simulink model "ugrid_hdetail_mod_linea_transmision"  (R2018a)
settings: Solver=VariableStepAuto  StartTime=0.0  StopTime=1  FixedStep=1e-6  MaxStep=1e-4  RelTol=1e-3
InitFcn:
  | SimulinkInit_linea_transmision
values from neighbouring files (symbols this model uses):
  b = 4.91    [SimulinkInit_linea_transmision.m]    (also in parametros_BIO.m; sistema.m = num(2))
  C = [C11; C22; C33;C44]    [Parametros_Sistema.m]    (also in SimulinkInit.m = 0.002654; SimulinkInit_linea_transmision.m = 1)
  C1 = 22e-6    (= 2.2e-05)    [Parametros_Sistema.m]    (also in SimulinkInit.m; SimulinkInit_linea_transmision.m; sistema.m)
  C2 = 22e-6    (= 2.2e-05)    [Parametros_Sistema.m]    (also in SimulinkInit.m; SimulinkInit_linea_transmision.m; sistema.m)
  C3 = 610e-6    (= 0.00061)    [Parametros_Sistema.m]    (also in SimulinkInit.m; SimulinkInit_linea_transmision.m; sistema.m)
  Cl = 20000e-6    (= 0.02)    [Parametros_Sistema.m]    (also in SimulinkInit.m = 0.002; SimulinkInit_linea_transmision.m; sistema.m)
  K = 25    [SimulinkInit_linea_transmision.m]    (also in parametros_BIO.m)
  K1 = 1.15    [SimulinkInit.m]    (also in SimulinkInit_linea_transmision.m = 9.66)
  K11 = 0.8    [SimulinkInit_linea_transmision.m]    (also in parametros_BIO.m)
  K2 = 1    [SimulinkInit.m]    (also in SimulinkInit_linea_transmision.m = 6.97)
  K22 = 0.2    [SimulinkInit_linea_transmision.m]    (also in parametros_BIO.m)
  K3 = 1    [SimulinkInit.m]    (also in SimulinkInit_linea_transmision.m = 31.8)
  K33 = 0.23    [SimulinkInit_linea_transmision.m]    (also in parametros_BIO.m)
  K4 = 15.1    [SimulinkInit_linea_transmision.m]    (also in parametros_BIO.m)
  Kd = 0.02    [SimulinkInit_linea_transmision.m]    (also in parametros_BIO.m)
  Kdc = 0.02    [SimulinkInit_linea_transmision.m]    (also in parametros_BIO.m)
  Kf = 1    [SimulinkInit_linea_transmision.m]    (also in parametros_BIO.m)
  Kh = 1.2    [SimulinkInit_linea_transmision.m]    (also in parametros_BIO.m)
  Ks = 21.5    [SimulinkInit_linea_transmision.m]    (also in parametros_BIO.m)
  Ksc = 3    [SimulinkInit_linea_transmision.m]    (also in parametros_BIO.m)
  Kv = 1    [SimulinkInit_linea_transmision.m]    (also in parametros_BIO.m)
  L = 5.2    [Parametros_Sistema.m]    (also in SimulinkInit_linea_transmision.m; sistema.m)
  L1 = 40e-3    (= 0.04)    [Parametros_Sistema.m]    (also in SimulinkInit.m; SimulinkInit_linea_transmision.m; sistema.m)
  L2 = 30e-3    (= 0.03)    [Parametros_Sistema.m]    (also in SimulinkInit.m = 0.005; SimulinkInit_linea_transmision.m; sistema.m)
  L3 = 5e-3    (= 0.005)    [Parametros_Sistema.m]    (also in SimulinkInit.m = 0.03; SimulinkInit_linea_transmision.m; sistema.m)
  L4 = 1e-3    (= 0.001)    [Parametros_Sistema.m]    (also in SimulinkInit.m = 5.2; SimulinkInit_linea_transmision.m = 3.5e-05; sistema.m)
  L5 = 10e-3    (= 0.01)    [Parametros_Sistema.m]    (also in SimulinkInit_linea_transmision.m = 2.2e-05; sistema.m)
  L6 = 40e-3    (= 0.04)    [Parametros_Sistema.m]    (also in SimulinkInit_linea_transmision.m = 1e-05; sistema.m)
  R = 10    [Parametros_Sistema.m]    (also in SimulinkInit_linea_transmision.m; sistema.m)
  R1 = 0.1    [Parametros_Sistema.m]    (also in SimulinkInit.m; SimulinkInit_linea_transmision.m; sistema.m)
  R2 = 0.2    [Parametros_Sistema.m]    (also in SimulinkInit.m = 0.1; SimulinkInit_linea_transmision.m; sistema.m)
  R3 = 1e-3    (= 0.001)    [Parametros_Sistema.m]    (also in SimulinkInit.m; SimulinkInit_linea_transmision.m; sistema.m)
  R4 = 10    [Parametros_Sistema.m]    (also in SimulinkInit.m; SimulinkInit_linea_transmision.m = 0.005; sistema.m)
  R5 = 4    [Parametros_Sistema.m]    (also in SimulinkInit.m = 10; SimulinkInit_linea_transmision.m = 0.0012; sistema.m)
  R6 = 25    [Parametros_Sistema.m]    (also in SimulinkInit_linea_transmision.m = 0.001; sistema.m)
  RL = 10    [Parametros_Sistema.m]    (also in SimulinkInit_linea_transmision.m; sistema.m)
  Sbin = 13.8    [SimulinkInit_linea_transmision.m]    (also in parametros_BIO.m)
  Svin = 2.91    [SimulinkInit_linea_transmision.m]    (also in parametros_BIO.m)
  T1 = 0.4    [SimulinkInit_linea_transmision.m]    (also in parametros_BIO.m)
  T2 = 1    [SimulinkInit_linea_transmision.m]    (also in parametros_BIO.m)
  T3 = 15    [SimulinkInit_linea_transmision.m]    (also in parametros_BIO.m)
  T4 = 2.5    [SimulinkInit_linea_transmision.m]    (also in parametros_BIO.m)
  T5 = 3.3    [SimulinkInit_linea_transmision.m]    (also in parametros_BIO.m)
  Tao1 = 0.5    [SimulinkInit.m]
  Tcd = 0.2    [SimulinkInit_linea_transmision.m]    (also in parametros_BIO.m)
  Tcr = 0.01    [SimulinkInit_linea_transmision.m]    (also in parametros_BIO.m)
  Tf = 0.04    [SimulinkInit_linea_transmision.m]    (also in parametros_BIO.m)
  Tr = 950    [SimulinkInit_linea_transmision.m]    (also in parametros_BIO.m)
  Tt = 450    [SimulinkInit_linea_transmision.m]    (also in parametros_BIO.m)
  Ttd = 0.04    [SimulinkInit_linea_transmision.m]    (also in parametros_BIO.m)
  Tv = 0.05    [SimulinkInit_linea_transmision.m]    (also in parametros_BIO.m)
  V = 20    [SimulinkInit_linea_transmision.m]    (also in parametros_BIO.m)
  wref = 70000    [SimulinkInit_linea_transmision.m]    (also in parametros_BIO.m)
  X_acid = 1.2    [SimulinkInit_linea_transmision.m]    (also in parametros_BIO.m)
  X_meth = 0.35    [SimulinkInit_linea_transmision.m]    (also in parametros_BIO.m)
  Z = 3    [SimulinkInit_linea_transmision.m]    (also in parametros_BIO.m)
undefined symbols (not defined in the file or in its folder): Ion, Lithium, sigbuilder_block, ss1, ss2
libraries: powerlib x64, dsparch4 x18, powerlib_meascontrol x4, simulink x1, mpclib x1, electricdrivelib x1
(part 2 of 2)

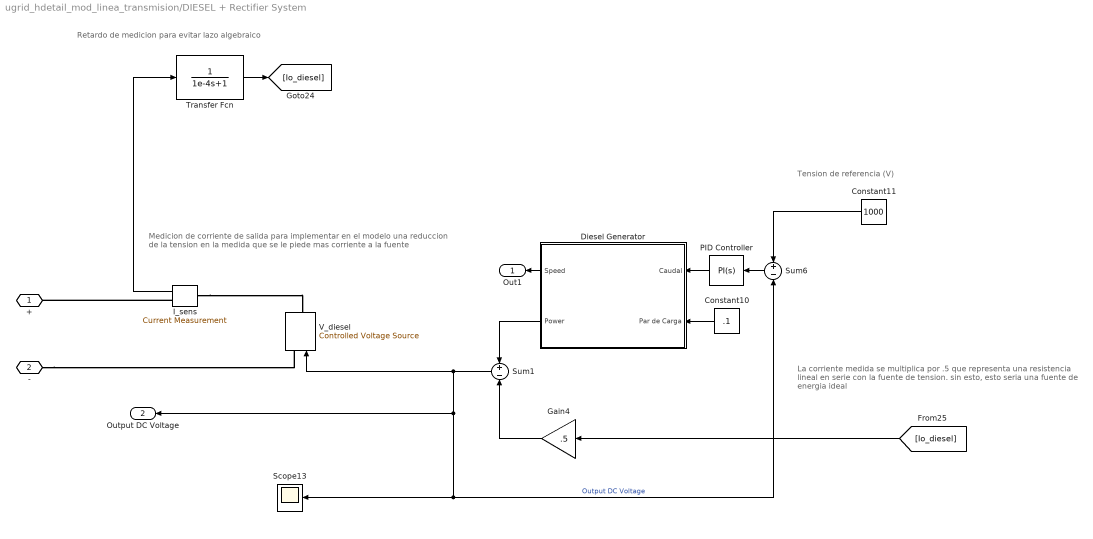
== system ugrid_hdetail_mod_linea_transmision/DIESEL + Rectifier System ==
  note: Tension de referencia (V)
  note: La corriente medida se multiplica por .5 que
      | representa una resistencia lineal en serie con
      | la fuente de tension. sin esto, esto seria una
      | fuente de energia ideal
  note: Medicion de corriente de salida para implementar
      | en el modelo una reduccion de la tension en la
      | medida que se le piede mas corriente a la fuente
  note: Retardo de medicion para evitar lazo algebraico
  Constant10 : Constant  Value=.1
  Constant11 : Constant  Value=1000
  Diesel Generator : Subsystem
  Gain4 : Gain  Gain=.5
  I_sens : powerlib/Measurements/Current Measurement  PhasorSimulation=off  OutputType=Complex  PSBequivalent=0
  PID Controller : simulink/Continuous/PID Controller  Controller=PI  TimeDomain=Continuous-time  SampleTime=-1  IntegratorMethod=Forward Euler  FilterMethod=Forward Euler  Form=Parallel  UseFilter=on  ControllerParametersSource=internal  P=0.00325909628031494  I=0.000326732379168699  D=0.00124823483730586  N=0.606508283225141  InitialConditionSource=internal  InitialConditionForIntegrator=0.248  InitialConditionForFilter=0.24  ExternalReset=none  LimitOutput=off  UpperSaturationLimit=inf  LowerSaturationLimit=-inf  LinearizeAsGain=on  AntiWindupMode=none  Kb=1  TrackingMode=off  Kt=1  PParamMin=[]  PParamMax=[]  IParamMin=[]  IParamMax=[]  DParamMin=[]  DParamMax=[]  NParamMin=[]  NParamMax=[]  KbParamMin=[]  KbParamMax=[]  KtParamMin=[]  KtParamMax=[]  POutMin=[]  POutMax=[]  IOutMin=[]  IOutMax=[]  DOutMin=[]  DOutMax=[]  NOutMin=[]  NOutMax=[]  KbOutMin=[]  KbOutMax=[]  KtOutMin=[]  KtOutMax=[]  IntegratorOutMin=[]  IntegratorOutMax=[]  FilterOutMin=[]  FilterOutMax=[]  SumOutMin=[]  SumOutMax=[]  SumI1OutMin=[]  SumI1OutMax=[]  SumI2OutMin=[]  SumI2OutMax=[]  SumI3OutMin=[]  SumI3OutMax=[]  SumDOutMin=[]  SumDOutMax=[]  SaturationOutMin=[]  SaturationOutMax=[]  IntegratorContinuousStateAttributes=''  IntegratorStateMustResolveToSignalObject=off  IntegratorRTWStateStorageClass=Auto  FilterContinuousStateAttributes=''  FilterStateMustResolveToSignalObject=off  FilterRTWStateStorageClass=Auto  DifferentiatorICPrevScaledInput=0  DifferentiatorOutMin=[]  DifferentiatorOutMax=[]  InitialConditionSetting=State (most efficient)  FilterDiffOutCoefMin=[]  FilterDiffOutCoefMax=[]  SumDenOutMin=[]  SumDenOutMax=[]  SumNumOutMin=[]  SumNumOutMax=[]  ReciprocalOutMin=[]  ReciprocalOutMax=[]  DivideOutMin=[]  DivideOutMax=[]  TunerSelectOption=Transfer Function Based (PID Tuner App)
  Scope13 : Scope
  Sum1 : Sum  Inputs=+-
  Sum6 : Sum  Inputs=+-
  Transfer Fcn : TransferFcn  Denominator=[1e-4 1]
  V_diesel : powerlib/Electrical Sources/Controlled Voltage Source  Initialize=on  Source_Type=AC  Amplitude=0  Phase=0  Frequency=0  Measurements=None
  + : PMIOPort  Side=Left
  - : PMIOPort  Port=2  Side=Left
  Out1 : Outport
  Output DC Voltage : Outport  Port=2
  wires:
  Sum1/1 -> Output DC Voltage/1, Sum6/2, Scope13/1, V_diesel/1  "Output DC Voltage"
  Transfer Fcn/1 -> [Io_diesel]
  I_sens/1 -> Transfer Fcn/1
  Diesel Generator/2(Power) -> Sum1/1
  Sum6/1 -> PID Controller/1
  Diesel Generator/1(Speed) -> Out1/1
  Gain4/1 -> Sum1/2
  Constant10/1 -> Diesel Generator/2(Par de Carga)
  Constant11/1 -> Sum6/1
  [Io_diesel] -> Gain4/1
  PID Controller/1 -> Diesel Generator/1(Caudal)
  connections:
  -/RConn1 -- V_diesel/LConn1
  I_sens/LConn1 -- V_diesel/RConn1
  I_sens/RConn1 -- +/RConn1

== system ugrid_hdetail_mod_linea_transmision/Signal Builder ==
  Demux : Demux  Tag=STV Demux  Outputs=1
  FromWs : FromWorkspace  Tag=STV FromWs  VariableName=tuvar  SampleTime=0
      SigBuilderData=|
      | common.afterFinalStr = 'Extrapolate'
      | common.sampleTime = 0
      | dataSet.timeRange = [0 10]
      | dataSet.name = 'Group 1'
      | sbobj.Groups.Name = 'Group 1'
      | sbobj.Groups.Signals.Name = 'Signal 1'
      | sbobj.Groups.Signals.XData = [0 0.1 0.1 0.2 0.2 0.3 0.3 0.4 0.4 0.5 0.5 0.6 0.6 0.7 0.7 0.8 0.8 0.9 0.9 10]
      | sbobj.Groups.Signals.YData = [0 0 500 500 1000 1000 1500 1500 2000 2000 2500 2500 3000 3000 3500 3500 4000 4000 4500 4500]
  Signal 1 : Outport  Tag=STV Outport
  wires:
  Demux/1 -> Signal 1/1
  FromWs/1 -> Demux/1

== system ugrid_hdetail_mod_linea_transmision/Signal Builder1 ==
  Demux : Demux  Tag=STV Demux  Outputs=1
  FromWs : FromWorkspace  Tag=STV FromWs  VariableName=tuvar  SampleTime=0
      SigBuilderData=|
      | common.afterFinalStr = 'Extrapolate'
      | common.sampleTime = 0
      | dataSet.timeRange = [0 10]
      | dataSet.name = 'Group 1'
      | sbobj.Groups.Name = 'Group 1'
      | sbobj.Groups.Signals.Name = 'Signal 1'
      | sbobj.Groups.Signals.XData = [0 0.1 0.1 0.4 0.4 0.8 0.8 10]
      | sbobj.Groups.Signals.YData = [0 0 100 100 200 200 500 500]
  Signal 1 : Outport  Tag=STV Outport
  wires:
  FromWs/1 -> Demux/1
  Demux/1 -> Signal 1/1

== system ugrid_hdetail_mod_linea_transmision/Signal Builder2 ==
  Demux : Demux  Tag=STV Demux  Outputs=1
  FromWs : FromWorkspace  Tag=STV FromWs  VariableName=tuvar  SampleTime=0
      SigBuilderData=|
      | common.afterFinalStr = 'Extrapolate'
      | common.sampleTime = 0
      | dataSet.timeRange = [0 10]
      | dataSet.name = 'Group 1'
      | sbobj.Groups.Name = 'Group 1'
      | sbobj.Groups.Signals.Name = 'Signal 1'
      | sbobj.Groups.Signals.XData = [0 0.1 0.1 0.2 0.2 0.3 0.3 0.4 0.4 0.5 0.5 0.6 0.6 0.7 0.7 0.8 0.8 0.9 0.9 10]
      | sbobj.Groups.Signals.YData = [0 0 500 500 1000 1000 1500 1500 2000 2000 2500 2500 3000 3000 3500 3500 4000 4000 4500 4500]
  Signal 1 : Outport  Tag=STV Outport
  wires:
  FromWs/1 -> Demux/1
  Demux/1 -> Signal 1/1

== system ugrid_hdetail_mod_linea_transmision/Signal Builder3 ==
  Demux : Demux  Tag=STV Demux  Outputs=1
  FromWs : FromWorkspace  Tag=STV FromWs  VariableName=tuvar  SampleTime=0
      SigBuilderData=|
      | common.afterFinalStr = 'Extrapolate'
      | common.sampleTime = 0
      | dataSet.timeRange = [0 10]
      | dataSet.name = 'Group 1'
      | sbobj.Groups.Name = 'Group 1'
      | sbobj.Groups.Signals.Name = 'Signal 1'
      | sbobj.Groups.Signals.XData = [0 0.1 0.1 0.4 0.4 0.8 0.8 10]
      | sbobj.Groups.Signals.YData = [0 0 100 100 200 200 500 500]
  Signal 1 : Outport  Tag=STV Outport
  wires:
  Demux/1 -> Signal 1/1
  FromWs/1 -> Demux/1

== system ugrid_hdetail_mod_linea_transmision/Subsystem ==
  Battery : electricdrivelib/Extra Sources/Battery  BatType=Lithium-Ion  ShowTempParam=off  ThermalPreset=no  ShowAgeParam=off  NomV=1000  NomQ=20  SOC=100  Batt_Tr=10e-3  PresetModel=off  MaxQ=1  MinV=825  FullV=1280.3859  Dis_rate=200  R=50e-3  Normal_OP=0.90435  expZone="[1188.4244    0.049130435]"  current=[6.5 13 32.5 50]  Units=Time  Tci=20  NomT=20  T2=-30  MaxQ2=4.8  FullV2=7.1  Normal_OP2=5.655  expZone2="[6.58           1]"  Rca=0.6  ti=2000  Dp=0  Neq0=0  Tsim=1e6  Ta1=25  Qeol=5.4*0.9  Reol=0.013333*1.2  Char_age=[2.3478, 3]  Dis_age=[2.3478, 10]  N1=1500  N2=10500  N3=1000  N4=1400  Ta2=45  N5=950
  Constant2 : Constant  Value=1000
  Constant4 : Constant  Value=25
  Controlled Current Source : powerlib/Electrical Sources/Controlled Current Source  Initialize=on  Source_Type=AC  Amplitude=0  Phase=0  Frequency=0  Measurements=None
  Gain3 : Gain  Gain=1/10
  PV panel1 : Subsystem
      mask Display: image('panel.jpg')
  Rcable : powerlib/Elements/Series RLC Branch  LConnTagsString=__new0  RConnTagsString=__new0  BranchType=R  Resistance=1e-3  Inductance=1e-3  SetiL0=off  InitialCurrent=0  Capacitance=1e-6  Setx0=off  InitialVoltage=0  Measurements=None
  Rin2 : powerlib/Elements/Series RLC Branch  LConnTagsString=__new0  RConnTagsString=__new0  BranchType=C  Resistance=.001  Inductance=0  SetiL0=off  InitialCurrent=0  Capacitance=1000e-6  Setx0=off  InitialVoltage=0  Measurements=None
  + : PMIOPort  Side=Left
  - : PMIOPort  Port=2  Side=Left
  Out1 : Outport
  wires:
  PV panel1/1(I) -> Gain3/1
  Gain3/1 -> Controlled Current Source/1
  Battery/1 -> Out1/1
  Constant4/1 -> PV panel1/3(Top)
  Constant2/1 -> PV panel1/2(G)
  [V] -> PV panel1/1(V)
  connections:
  Rcable/RConn1 -- +/RConn1
  Battery/LConn1 -- Controlled Current Source/RConn1 -- Rcable/LConn1 -- Rin2/LConn1
  Battery/LConn2 -- -/RConn1 -- Rin2/RConn1 -- Controlled Current Source/LConn1

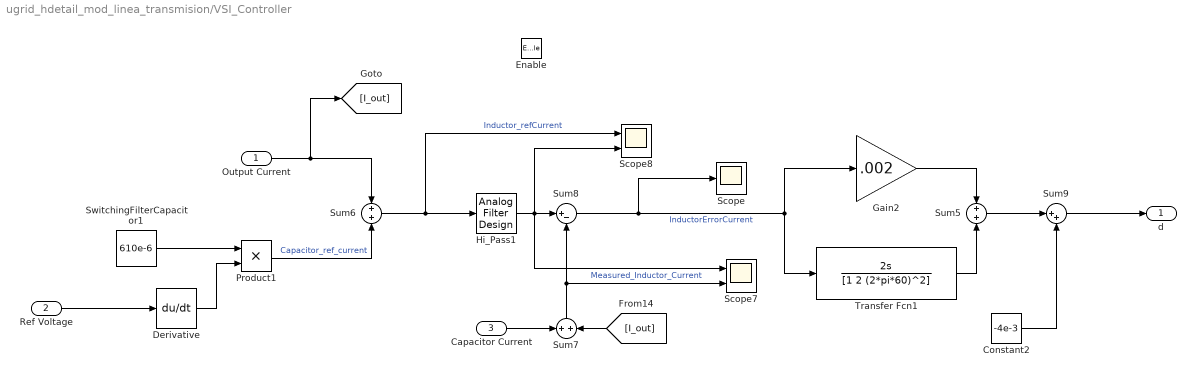
== system ugrid_hdetail_mod_linea_transmision/VSI_Controller ==
  Output Current : Inport
  Ref Voltage : Inport  Port=2
  Capacitor Current : Inport  Port=3
  Enable : EnablePort
  Constant2 : Constant  Value=-4e-3
  Derivative : Derivative  CoefficientInTFapproximation=1e-3
  Gain2 : Gain  Gain=.002
  Hi_Pass1 : dsparch4/Analog Filter Design  method=Bessel  filttype=Highpass  N=1  Wlo=1*2*pi  Whi=80  Rp=2  Rs=40
  Product1 : Product
  Scope : Scope
  Scope7 : Scope  NumInputPorts=2
  Scope8 : Scope  NumInputPorts=2
  Sum5 : Sum  Inputs=+|+
  Sum6 : Sum  Inputs=+|+
  Sum7 : Sum  Inputs=+|+
  Sum8 : Sum  Inputs=|+-
  Sum9 : Sum  Inputs=|++
  SwitchingFilterCapacitor1 : Constant  Value=610e-6
  Transfer Fcn1 : TransferFcn  Numerator=[2 0]  Denominator=[1 2 (2*pi*60)^2]
  d : Outport
  wires:
  Derivative/1 -> Product1/2
  Sum6/1 -> Hi_Pass1/1, Scope8/1  "Inductor_refCurrent"
  Sum8/1 -> Scope/1, Transfer Fcn1/1, Gain2/1  "InductorErrorCurrent"
  Ref Voltage/1 -> Derivative/1
  Constant2/1 -> Sum9/2
  Capacitor Current/1 -> Sum7/1
  Transfer Fcn1/1 -> Sum5/2
  Output Current/1 -> Sum6/1, [I_out]
  [I_out] -> Sum7/2
  Gain2/1 -> Sum5/1
  SwitchingFilterCapacitor1/1 -> Product1/1
  Hi_Pass1/1 -> Scope8/2, Sum8/1, Scope7/1
  Product1/1 -> Sum6/2  "Capacitor_ref_current"
  Sum9/1 -> d/1
  Sum5/1 -> Sum9/1
  Sum7/1 -> Scope7/2, Sum8/2  "Measured_Inductor_Current"

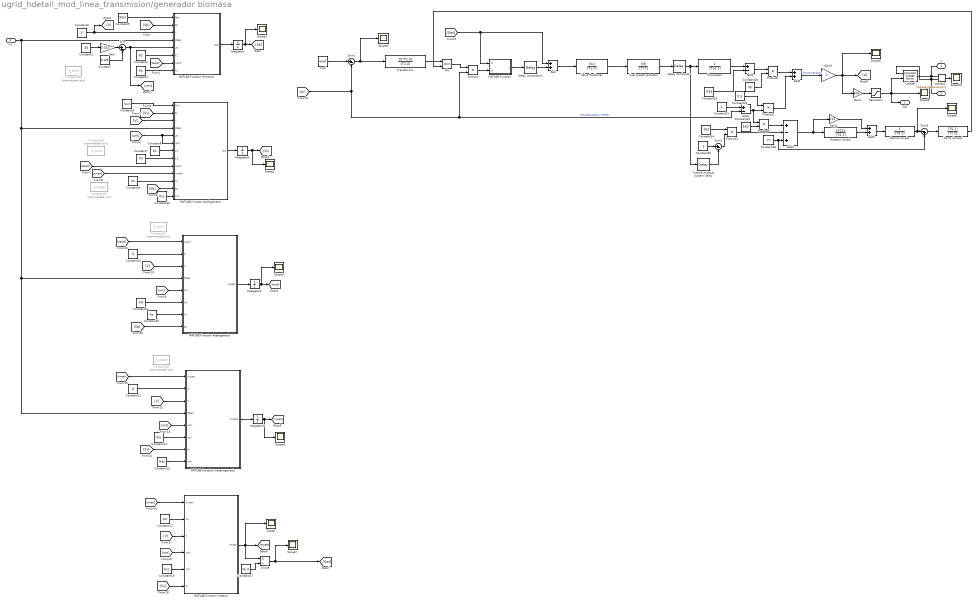
== system ugrid_hdetail_mod_linea_transmision/generador biomasa ==
  In1 : Inport
  Add : Sum
  Add1 : Sum  Inputs=+-
  Add2 : Sum
  Add3 : Sum  Inputs=+-
  Add4 : Sum  Inputs=+-+
  Add5 : Sum
  Compresor : TransferFcn  Denominator=[Tcd 1]
  Constant : Constant  Value=0.129
  Constant1 : Constant  Value=35
  Constant10 : Constant  Value=Ksc
  Constant11 : Constant  Value=b
  Constant12 : Constant  Value=b
  Constant13 : Constant  Value=Kdc
  Constant14 : Constant  Value=Ksc
  Constant15 : Constant  Value=Ks
  Constant16 : Constant  Value=Kd
  Constant17 : Constant  Value=K4
  Constant18 : Constant  Value=Ksc
  Constant19 : Constant  Value=K33
  Constant2 : Constant  Value=Ks
  Constant20 : Constant  Value=Kh
  Constant21 : Constant
  Constant22 : Constant  Value=0.5
  Constant23 : Constant  Value=550
  Constant24 : Constant  Value=700
  Constant25 : Constant
  Constant26 : Constant  Value=Tr
  Constant27 : Constant  Value=35.4
  Constant28 : Constant  Commented=on  Value=X_acid
  Constant29 : Constant  Commented=on  Value=X_acid
  Constant3 : Constant  Value=V
  Constant30 : Constant  Commented=on  Value=X_meth
  Constant31 : Constant  Commented=on  Value=X_acid
  Constant32 : Constant  Commented=on  Value=X_meth
  Constant4 : Constant  Value=K1
  Constant5 : Constant  Value=Sbin
  Constant6 : Constant  Value=Svin
  Constant7 : Constant  Value=K3
  Constant8 : Constant  Value=K2
  Constant9 : Constant  Value=Ks
  Delay combustor : TransportDelay  DelayTime=Tcr
  Delay combustor1 : TransportDelay  DelayTime=0
  Divide : Product  Inputs=*/
  Fuel system actuator : TransferFcn  Numerator=[Kf]  Denominator=[Tf C]
  Gain : Gain  Gain=0.013
  Gain1 : Gain  Gain=900
  Gain2 : Gain  Gain=K11
  Gain3 : Gain
  Integrator : Integrator
  Integrator1 : Integrator
  Integrator2 : Integrator  InitialCondition=1.2
  Integrator3 : Integrator  InitialCondition=0.35
  MATLAB Function : MATLAB Function  TreatAsAtomicUnit=on
  MATLAB Function Acetogenesis : MATLAB Function  TreatAsAtomicUnit=on
  MATLAB Function Acidogenesis : MATLAB Function  TreatAsAtomicUnit=on
  MATLAB Function Hidrolisis : MATLAB Function  TreatAsAtomicUnit=on
  MATLAB Function metano : MATLAB Function  TreatAsAtomicUnit=on
  MATLAB Function metanogenesis : MATLAB Function  TreatAsAtomicUnit=on
  Min : MinMax  Inputs=2
  Product{,1..4} (5 alike) : Product
  Rotation Shield : TransferFcn  Numerator=[K22]  Denominator=[T3 1]
  Saturation : Saturate  UpperLimit=1000  LowerLimit=0
  Scope{,1..10} (11 alike) : Scope
  Sum : Sum  Inputs=|+-
  Sum1 : Sum  Inputs=|+-
  Sum2 : Sum  Inputs=|+-
  Sum3 : Sum  Inputs=|-+
  Temp Control : TransferFcn  Numerator=[T5 1]  Denominator=[Tt 0]
  Transfer Fcn : TransferFcn  Numerator=[K*T1 K]  Denominator=[T2 Z]
  Turbine exhaust system delay : TransportDelay  DelayTime=Ttd
  V_diesel : powerlib/Electrical Sources/Controlled Voltage Source  Initialize=on  Source_Type=DC  Amplitude=0  Phase=0  Frequency=0  Measurements=None
  Valve Positioner : TransferFcn  Numerator=[Kv]  Denominator=[Tv C]
  Vsensa1 : powerlib/Measurements/Voltage Measurement  PhasorSimulation=off  OutputType=Complex  PSBequivalent=0
  thermo couple : TransferFcn  Denominator=[T4 1]
  wref : Constant  Value=wref
  + : PMIOPort  Side=Left
  - : PMIOPort  Port=2  Side=Left
  Vdc : Outport
  wires:
  MATLAB Function metano/1(Fmeth) -> Divide/1, Scope/1, [Fmeth]
  Sum/1 -> [um], MATLAB Function Hidrolisis/5(um)
  Constant16/1 -> MATLAB Function Acetogenesis/6(Kd)
  Temp Control/1 -> Min/2
  Integrator/1 -> Scope1/1, [Sb]
  Gain3/1 -> Gain1/1, Scope5/1, [w]
  Sum1/1 -> Transfer Fcn/1, Scope6/1
  [Sb] -> MATLAB Function Acetogenesis/8(Sb)
  [Sv] -> MATLAB Function metanogenesis/7(Sv)
  Add4/1 -> Rotation Shield/1, Gain2/1
  Constant8/1 -> MATLAB Function Acidogenesis/7(K2)
  Constant24/1 -> Product4/1
  [V] -> MATLAB Function Acetogenesis/3(V)
  Constant23/1 -> Product3/2
  Constant27/1 -> Divide/2
  [Sb] -> MATLAB Function Acidogenesis/12(Sb)
  Integrator3/1 -> Scope4/1, [Xmeth]
  Integrator2/1 -> Scope3/1, [Xacid]
  Divide/1 -> Scope7/1, [Gas]
  Constant7/1 -> MATLAB Function Acidogenesis/8(K3)
  Delay combustor/1 -> Turbine exhaust system delay/1, Compresor/1
  [V] -> MATLAB Function Acidogenesis/3(V)
  Constant12/1 -> MATLAB Function Acetogenesis/2(b)
  Sum2/1 -> Product4/2
  [V] -> MATLAB Function metanogenesis/3(V)
  Gain/1 -> Sum/1
  Product/1 -> MATLAB Function/2(u2)
  [w] -> Product/2, Add3/2, Sum1/2  "velocidad angular medida"
  Constant6/1 -> MATLAB Function Acidogenesis/1(Svin)
  wref/1 -> Sum1/1
  [Gas] -> MATLAB Function/1(u1), Add/1
  [Sv] -> MATLAB Function metano/6(Sv)
  MATLAB Function Hidrolisis/1(Sbp) -> Integrator/1
  Turbine exhaust system delay/1 -> Sum2/2
  MATLAB Function Acetogenesis/1(Xacidp) -> Integrator2/1
  Constant/1 -> Sum/2
  Constant18/1 -> MATLAB Function metano/5(Ksc)
  In1/1 -> MATLAB Function Acidogenesis/4(Ffeed), MATLAB Function metanogenesis/4(Ffeed), MATLAB Function Acetogenesis/4(Ffeed), MATLAB Function Hidrolisis/4(Ffeed)
  Add3/1 -> Product3/1, Product2/2
  [um] -> MATLAB Function Acetogenesis/5(um)
  Product3/1 -> Add4/1
  Constant15/1 -> MATLAB Function Acetogenesis/7(Ks)
  thermo couple/1 -> Scope8/1, Sum3/1
  Fuel system actuator/1 -> Delay combustor/1
  Add/1 -> Valve Positioner/1
  Add5/1 -> thermo couple/1
  Gain2/1 -> Add5/1
  Constant22/1 -> Product2/1
  [um] -> MATLAB Function metano/4(umc)
  Compresor/1 -> Add1/1
  Constant10/1 -> MATLAB Function Acidogenesis/13(Ksc)
  [um] -> MATLAB Function Acidogenesis/6(umc), MATLAB Function Acidogenesis/5(um)
  Constant9/1 -> MATLAB Function Acidogenesis/11(Ks)
  Constant1/1 -> Gain/1
  Constant13/1 -> MATLAB Function metanogenesis/8(Kdc)
  Constant26/1 -> Sum3/2, Add4/3
  Integrator1/1 -> Scope2/1, [Sv]
  [Xmeth] -> MATLAB Function metanogenesis/1(Xmeth)
  Add2/1 -> Gain3/1  "Torque mecánico"
  MATLAB Function/1(y) -> Delay combustor1/1
  Saturation/1 -> Vdc/1, V_diesel/1, Scope9/1
  [Sb] -> MATLAB Function Hidrolisis/2(Sb)
  Min/1 -> Product/1
  Constant3/1 -> [V], MATLAB Function Hidrolisis/3(V)
  MATLAB Function Acidogenesis/1(Svp) -> Integrator1/1
  Constant5/1 -> MATLAB Function Hidrolisis/1(Sbin)
  Constant20/1 -> Product1/2
  [Xmeth] -> MATLAB Function Acidogenesis/10(Xmeth)
  Sum3/1 -> Temp Control/1
  Gain1/1 -> Saturation/1
  Constant21/1 -> Add3/1
  Constant25/1 -> Sum2/1
  Product2/1 -> Add2/2
  [Xacid] -> MATLAB Function Acidogenesis/9(Xacid)
  Valve Positioner/1 -> Fuel system actuator/1
  Constant4/1 -> MATLAB Function Hidrolisis/6(K1)
  Constant11/1 -> MATLAB Function metanogenesis/2(b)
  Rotation Shield/1 -> Add5/2
  Add1/1 -> Product1/1
  [Sv] -> MATLAB Function Acidogenesis/2(Sv)
  [Xacid] -> MATLAB Function Acetogenesis/1(Xacid)
  Constant19/1 -> Add1/2
  Product1/1 -> Add2/1
  Transfer Fcn/1 -> Min/1
  Delay combustor1/1 -> Add/2
  [um] -> MATLAB Function metanogenesis/5(umc)
  MATLAB Function metanogenesis/1(Xmethp) -> Integrator3/1
  Constant14/1 -> MATLAB Function metanogenesis/6(Ksc)
  Product4/1 -> Add4/2
  Constant2/1 -> MATLAB Function Hidrolisis/8(Ks)
  Constant17/1 -> MATLAB Function metano/2(K4)
  [V] -> MATLAB Function metano/3(V)
  [Xmeth] -> MATLAB Function metano/1(Xmeth)
  [Xacid] -> MATLAB Function Hidrolisis/7(Xacid)
  Vsensa1/1 -> Scope10/1
  connections:
  V_diesel/RConn1 -- Vsensa1/LConn1 -- +/RConn1
  V_diesel/LConn1 -- Vsensa1/LConn2 -- -/RConn1

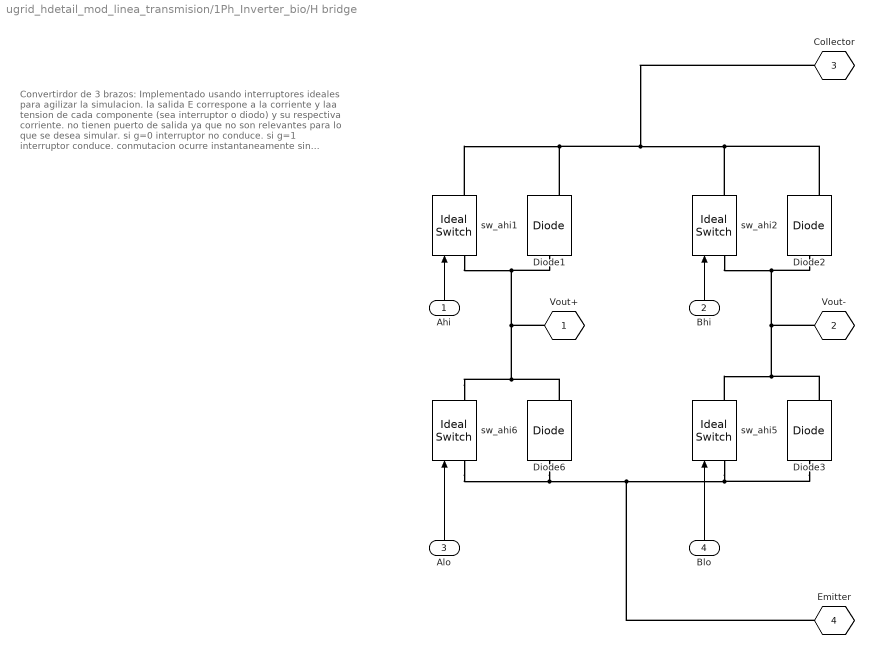
== system ugrid_hdetail_mod_linea_transmision/1Ph_Inverter_bio/H bridge ==
  note: Convertirdor de 3 brazos:
      |
      | Implementado usando interruptores
      | ideales para agilizar la simulacion.
      | la salida E correspone a la corriente y laa
      | tension de cada componente
      | (sea interruptor o diodo) y su respectiva
      | corriente. no tienen puerto de salida ya que no
      | son relevantes para lo que se desea simular.
      |
      | si g=0 interruptor no conduce.
      | si g=1 interruptor conduce.
      |
      | conmutacion ocurre instantaneamente sin
      | retardo.
  Ahi : Inport
  Bhi : Inport  Port=2
  Alo : Inport  Port=3
  Blo : Inport  Port=4
   sw_ahi{1..2,5..6} (4 alike) : powerlib/Power Electronics/Ideal Switch  Ron=0.1  Lon=0  IC=0  Rs=1e6  Cs=10e-12  Measurements=on
  Diode{1..3,6} (4 alike) : powerlib/Power Electronics/Diode  Ron=.2  Lon=0  Vf=0.8  IC=0  UseSnubber=0  Rs=0  Cs=0  Measurements=on
  " Vout+" : PMIOPort  Tag=PMCPort  Side=Right
  Vout- : PMIOPort  Tag=PMCPort  Port=2  Side=Right
  Collector : PMIOPort  Tag=PMCPort  Port=3  Side=Right
  Emitter : PMIOPort  Tag=PMCPort  Port=4  Side=Right
  wires:
  Alo/1 -> " sw_ahi6"/1
  Ahi/1 -> " sw_ahi1"/1
  Blo/1 -> " sw_ahi5"/1
  Bhi/1 -> " sw_ahi2"/1
  connections:
  Diode3/RConn1 -- Vout-/RConn1 -- " sw_ahi2"/LConn1 -- Diode2/LConn1 -- " sw_ahi5"/RConn1
  Diode3/LConn1 -- Emitter/RConn1 -- Diode6/LConn1 -- " sw_ahi6"/LConn1 -- " sw_ahi5"/LConn1
  Diode2/RConn1 -- Collector/RConn1 -- " sw_ahi1"/RConn1 -- Diode1/RConn1 -- " sw_ahi2"/RConn1
  " sw_ahi6"/RConn1 -- Diode6/RConn1 -- " Vout+"/RConn1 -- Diode1/LConn1 -- " sw_ahi1"/LConn1

== system ugrid_hdetail_mod_linea_transmision/1Ph_Inverter_bio/Io_measure ==
  A_current : Inport
  Enable : EnablePort
  Hw1 : dsparch4/Analog Filter Design  method=Bessel  filttype=Lowpass  N=2  Wlo=7000*2*pi  Whi=80  Rp=2  Rs=80
  Transfer Fcn : TransferFcn  Denominator=[1e-6 1]
  Out1 : Outport
  wires:
  Transfer Fcn/1 -> Hw1/1
  A_current/1 -> Transfer Fcn/1
  Hw1/1 -> Out1/1

== system ugrid_hdetail_mod_linea_transmision/1Ph_Inverter_bio/Subsystem ==
  Din : Inport
  Enable : EnablePort
  Gain : Gain  Gain=15
  PWM Generator (DC-DC) : powerlib_meascontrol/Pulse & Signal Generators/PWM Generator (DC-DC)  Fsw=f_sw  Ts=samp_f
  Steper1 : Subsystem
  Steper3 : Subsystem
  not_pwm : MATLAB Function  TreatAsAtomicUnit=on
  nPWM : Outport
  PWM : Outport  Port=2
  wires:
  not_pwm/1(y) -> Steper3/1(In1)
  Steper3/1(Out1) -> nPWM/1
  Gain/1 -> Steper1/1(In1), not_pwm/1(u)
  Din/1 -> PWM Generator (DC-DC)/1
  PWM Generator (DC-DC)/1 -> Gain/1
  Steper1/1(Out1) -> PWM/1

== system ugrid_hdetail_mod_linea_transmision/1Ph_Inverter_bio/Subsystem1 ==
  A_volts : Inport
  Enable : EnablePort
  Hw4 : dsparch4/Analog Filter Design  method=Bessel  filttype=Lowpass  N=2  Wlo=7000*2*pi  Whi=80  Rp=2  Rs=80
  Transfer Fcn1 : TransferFcn  Denominator=[1e-6 1]
  Out1 : Outport
  wires:
  A_volts/1 -> Transfer Fcn1/1
  Transfer Fcn1/1 -> Hw4/1
  Hw4/1 -> Out1/1

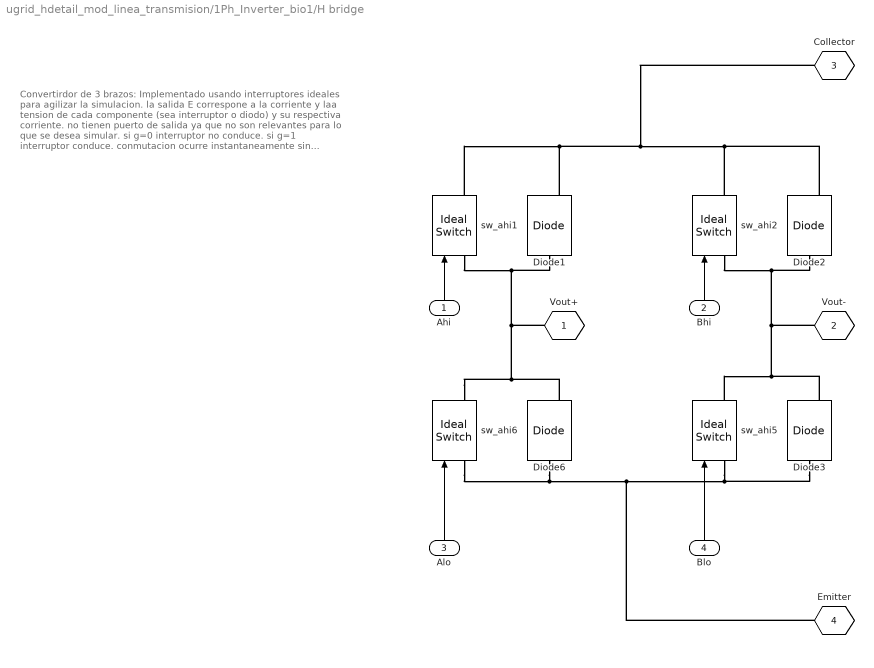
== system ugrid_hdetail_mod_linea_transmision/1Ph_Inverter_bio1/H bridge ==
  note: Convertirdor de 3 brazos:
      |
      | Implementado usando interruptores
      | ideales para agilizar la simulacion.
      | la salida E correspone a la corriente y laa
      | tension de cada componente
      | (sea interruptor o diodo) y su respectiva
      | corriente. no tienen puerto de salida ya que no
      | son relevantes para lo que se desea simular.
      |
      | si g=0 interruptor no conduce.
      | si g=1 interruptor conduce.
      |
      | conmutacion ocurre instantaneamente sin
      | retardo.
  Ahi : Inport
  Bhi : Inport  Port=2
  Alo : Inport  Port=3
  Blo : Inport  Port=4
   sw_ahi{1..2,5..6} (4 alike) : powerlib/Power Electronics/Ideal Switch  Ron=0.1  Lon=0  IC=0  Rs=1e6  Cs=10e-12  Measurements=on
  Diode{1..3,6} (4 alike) : powerlib/Power Electronics/Diode  Ron=.2  Lon=0  Vf=0.8  IC=0  UseSnubber=0  Rs=0  Cs=0  Measurements=on
  " Vout+" : PMIOPort  Tag=PMCPort  Side=Right
  Vout- : PMIOPort  Tag=PMCPort  Port=2  Side=Right
  Collector : PMIOPort  Tag=PMCPort  Port=3  Side=Right
  Emitter : PMIOPort  Tag=PMCPort  Port=4  Side=Right
  wires:
  Alo/1 -> " sw_ahi6"/1
  Ahi/1 -> " sw_ahi1"/1
  Blo/1 -> " sw_ahi5"/1
  Bhi/1 -> " sw_ahi2"/1
  connections:
  Diode3/RConn1 -- Vout-/RConn1 -- " sw_ahi2"/LConn1 -- Diode2/LConn1 -- " sw_ahi5"/RConn1
  Diode3/LConn1 -- Emitter/RConn1 -- Diode6/LConn1 -- " sw_ahi6"/LConn1 -- " sw_ahi5"/LConn1
  Diode2/RConn1 -- Collector/RConn1 -- " sw_ahi1"/RConn1 -- Diode1/RConn1 -- " sw_ahi2"/RConn1
  " sw_ahi6"/RConn1 -- Diode6/RConn1 -- " Vout+"/RConn1 -- Diode1/LConn1 -- " sw_ahi1"/LConn1

== system ugrid_hdetail_mod_linea_transmision/1Ph_Inverter_bio1/Ic Measure ==
  Ic : Inport
  Enable : EnablePort
  Hw5 : dsparch4/Analog Filter Design  method=Bessel  filttype=Lowpass  N=2  Wlo=7000*2*pi  Whi=80  Rp=2  Rs=80
  Transfer Fcn2 : TransferFcn  Denominator=[1e-6 1]
  Out1 : Outport
  wires:
  Transfer Fcn2/1 -> Hw5/1
  Ic/1 -> Transfer Fcn2/1
  Hw5/1 -> Out1/1

== system ugrid_hdetail_mod_linea_transmision/1Ph_Inverter_bio1/Io_measure ==
  A_current : Inport
  Enable : EnablePort
  Hw2 : dsparch4/Analog Filter Design  method=Bessel  filttype=Lowpass  N=2  Wlo=7000*2*pi  Whi=80  Rp=2  Rs=80
  Transfer Fcn : TransferFcn  Denominator=[1e-6 1]
  Out1 : Outport
  wires:
  Transfer Fcn/1 -> Hw2/1
  Hw2/1 -> Out1/1
  A_current/1 -> Transfer Fcn/1

== system ugrid_hdetail_mod_linea_transmision/1Ph_Inverter_bio1/Steper1 ==
  In1 : Inport
  Product : Product
  Step : Step  Time=st_time  SampleTime=samp_f
  Out1 : Outport
  wires:
  Step/1 -> Product/2
  In1/1 -> Product/1
  Product/1 -> Out1/1

== system ugrid_hdetail_mod_linea_transmision/1Ph_Inverter_bio1/Steper3 ==
  In1 : Inport
  Product : Product
  Step : Step  Time=st_time  SampleTime=samp_f
  Out1 : Outport
  wires:
  Product/1 -> Out1/1
  In1/1 -> Product/1
  Step/1 -> Product/2

== system ugrid_hdetail_mod_linea_transmision/1Ph_Inverter_bio1/Vo_measure ==
  A_volts : Inport
  Enable : EnablePort
  Hw6 : dsparch4/Analog Filter Design  method=Bessel  filttype=Lowpass  N=2  Wlo=7000*2*pi  Whi=80  Rp=2  Rs=80
  Transfer Fcn1 : TransferFcn  Denominator=[1e-6 1]
  Out1 : Outport
  wires:
  Transfer Fcn1/1 -> Hw6/1
  Hw6/1 -> Out1/1
  A_volts/1 -> Transfer Fcn1/1

== system ugrid_hdetail_mod_linea_transmision/1Ph_Inverter_diesel/H bridge ==
  note: Convertirdor de 3 brazos:
      |
      | Implementado usando interruptores
      | ideales para agilizar la simulacion.
      | la salida E correspone a la corriente y laa
      | tension de cada componente
      | (sea interruptor o diodo) y su respectiva
      | corriente. no tienen puerto de salida ya que no
      | son relevantes para lo que se desea simular.
      |
      | si g=0 interruptor no conduce.
      | si g=1 interruptor conduce.
      |
      | conmutacion ocurre instantaneamente sin
      | retardo.
  Ahi : Inport
  Bhi : Inport  Port=2
  Alo : Inport  Port=3
  Blo : Inport  Port=4
   sw_ahi{1..2,5..6} (4 alike) : powerlib/Power Electronics/Ideal Switch  Ron=0.1  Lon=0  IC=0  Rs=1e6  Cs=10e-12  Measurements=on
  Diode{1..3,6} (4 alike) : powerlib/Power Electronics/Diode  Ron=.2  Lon=0  Vf=0.8  IC=0  UseSnubber=0  Rs=0  Cs=0  Measurements=on
  " Vout+" : PMIOPort  Tag=PMCPort  Side=Right
  Vout- : PMIOPort  Tag=PMCPort  Port=2  Side=Right
  Collector : PMIOPort  Tag=PMCPort  Port=3  Side=Right
  Emitter : PMIOPort  Tag=PMCPort  Port=4  Side=Right
  wires:
  Bhi/1 -> " sw_ahi2"/1
  Blo/1 -> " sw_ahi5"/1
  Ahi/1 -> " sw_ahi1"/1
  Alo/1 -> " sw_ahi6"/1
  connections:
  " sw_ahi1"/LConn1 -- Diode1/LConn1 -- " Vout+"/RConn1 -- Diode6/RConn1 -- " sw_ahi6"/RConn1
  " sw_ahi2"/RConn1 -- Diode1/RConn1 -- " sw_ahi1"/RConn1 -- Collector/RConn1 -- Diode2/RConn1
  " sw_ahi5"/LConn1 -- " sw_ahi6"/LConn1 -- Diode6/LConn1 -- Emitter/RConn1 -- Diode3/LConn1
  " sw_ahi5"/RConn1 -- Diode2/LConn1 -- " sw_ahi2"/LConn1 -- Vout-/RConn1 -- Diode3/RConn1

== system ugrid_hdetail_mod_linea_transmision/1Ph_Inverter_diesel/Io_measure ==
  A_current : Inport
  Enable : EnablePort
  Hw7 : dsparch4/Analog Filter Design  method=Bessel  filttype=Lowpass  N=2  Wlo=7000*2*pi  Whi=80  Rp=2  Rs=80
  Transfer Fcn : TransferFcn  Denominator=[1e-6 1]
  Out1 : Outport
  wires:
  Hw7/1 -> Out1/1
  Transfer Fcn/1 -> Hw7/1
  A_current/1 -> Transfer Fcn/1

== system ugrid_hdetail_mod_linea_transmision/1Ph_Inverter_diesel/Subsystem ==
  Din : Inport
  Enable : EnablePort
  Gain : Gain  Gain=15
  PWM Generator (DC-DC) : powerlib_meascontrol/Pulse & Signal Generators/PWM Generator (DC-DC)  Fsw=f_sw  Ts=samp_f
  Steper1 : Subsystem
  Steper3 : Subsystem
  not_pwm : MATLAB Function  TreatAsAtomicUnit=on
  nPWM : Outport
  PWM : Outport  Port=2
  wires:
  PWM Generator (DC-DC)/1 -> Gain/1
  Gain/1 -> not_pwm/1(u), Steper1/1(In1)
  Din/1 -> PWM Generator (DC-DC)/1
  not_pwm/1(y) -> Steper3/1(In1)
  Steper3/1(Out1) -> nPWM/1
  Steper1/1(Out1) -> PWM/1

== system ugrid_hdetail_mod_linea_transmision/1Ph_Inverter_diesel/Vo_measure ==
  A_volts : Inport
  Enable : EnablePort
  Hw3 : dsparch4/Analog Filter Design  method=Bessel  filttype=Lowpass  N=2  Wlo=7000*2*pi  Whi=80  Rp=2  Rs=80
  Transfer Fcn1 : TransferFcn  Denominator=[1e-6 1]
  Out1 : Outport
  wires:
  Transfer Fcn1/1 -> Hw3/1
  Hw3/1 -> Out1/1
  A_volts/1 -> Transfer Fcn1/1

== system ugrid_hdetail_mod_linea_transmision/CSI_Control_BIO/PR Controller_0_ref 3 ==
  ref : Inport
  real : Inport  Port=2
  K1 : Gain  Gain=Kp
  K2 : Gain  Gain=Ki
  Scope : Scope
  Steper6 : Subsystem
  Sum : Sum  Inputs=+-
  Sum1 : Sum  Inputs=+|+
  Transfer Fcn : TransferFcn  Numerator=[1 0]  Denominator=[1 wa (w0)^2]
  Out1 : Outport
  wires:
  real/1 -> Sum/2
  ref/1 -> Sum/1
  Sum/1 -> Scope/1, Steper6/1(In1)  "error en pr bio"
  K1/1 -> Sum1/1
  Transfer Fcn/1 -> Sum1/2
  K2/1 -> Transfer Fcn/1
  Steper6/1(Out1) -> K1/1, K2/1
  Sum1/1 -> Out1/1

== system ugrid_hdetail_mod_linea_transmision/CSI_Control_DIESEL/PR Controller_0_ref 3 ==
  ref : Inport
  real : Inport  Port=2
  K1 : Gain  Gain=Kp
  K2 : Gain  Gain=Ki
  Scope : Scope
  Steper6 : Subsystem
  Sum : Sum  Inputs=+-
  Sum1 : Sum  Inputs=+|+
  Transfer Fcn : TransferFcn  Numerator=[1 0]  Denominator=[1 wa (w0)^2]
  Out1 : Outport
  wires:
  Sum1/1 -> Out1/1
  Steper6/1(Out1) -> K2/1, K1/1
  K2/1 -> Transfer Fcn/1
  Transfer Fcn/1 -> Sum1/2
  K1/1 -> Sum1/1
  Sum/1 -> Scope/1, Steper6/1(In1)  "error pr gen"
  ref/1 -> Sum/1
  real/1 -> Sum/2

== system ugrid_hdetail_mod_linea_transmision/DIESEL + Rectifier System/Diesel Generator ==
  Caudal : Inport
  Par de Carga : Inport  Port=2
  " 1" : Gain  Gain=1.15
  " Generador1" : Gain  Gain=1/2
  Gain1 : Gain  Gain=12000
  Motor de Combustión1 : TransportDelay  DelayTime=Tao1
  Scope : Scope
  State-Space : StateSpace  A=ss1.A  B=ss1.B  C=ss1.C  D=ss1.D  InitialCondition=0.17566/ss1.C
  State-Space1 : StateSpace  A=ss2.A  B=ss2.B  C=ss2.C  D=ss2.D  InitialCondition=0.2493/ss2.C
  Sum2 : Sum  Inputs=|+-
  Speed : Outport
  Power : Outport  Port=2
  wires:
  " 1"/1 -> Motor de Combustión1/1
  " Generador1"/1 -> Gain1/1
  Motor de Combustión1/1 -> Sum2/1
  State-Space1/1 -> Scope/1, " 1"/1
  State-Space/1 -> Speed/1, " Generador1"/1  "Velocidad"
  Sum2/1 -> State-Space/1
  Caudal/1 -> State-Space1/1
  Par de Carga/1 -> Sum2/2
  Gain1/1 -> Power/1

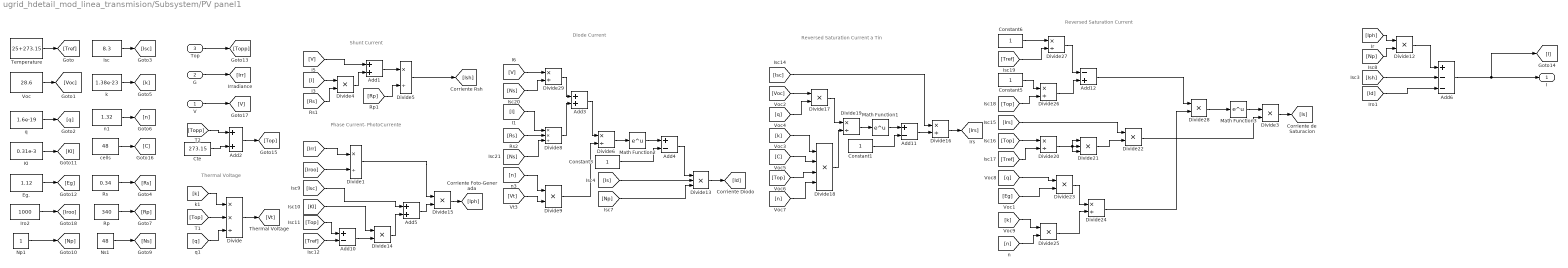
== system ugrid_hdetail_mod_linea_transmision/Subsystem/PV panel1 ==
  note: Thermal Voltage
  note: Shunt Current
  note: Phase Current- PhotoCurrente
  note: Diode Current
  note: Reversed Saturation Current a Tin
  note: Reversed Saturation Current
  V : Inport
  G : Inport  Port=2
  Top : Inport  Port=3
  Add{1..3,5} (4 alike) : Sum
  Add10 : Sum  Inputs=+-
  Add11 : Sum  Inputs=+-
  Add12 : Sum  Inputs=-+
  Add4 : Sum  Inputs=+-
  Add6 : Sum  Inputs=+--
  Constant{1,3,5..6} (4 alike) : Constant
  Cte : Constant  Value=273.15
  Divide : Product  Inputs=**/
  Divide{1,5..6,16,19..20,24,26..27,29} (10 alike) : Product  Inputs=*/
  Divide{3..4,9,12,14..15,17,22..23,25,28} (11 alike) : Product  Inputs=**
  Divide13 : Product  Inputs=***
  Divide18 : Product  Inputs=****
  Divide21 : Product  Inputs=***
  Divide8 : Product  Inputs=**/
  Eg. : Constant  Value=1.12
  Iro2 : Constant  Value=1000
  Isc : Constant  Value=8.3
  KI : Constant  Value=0.31e-3
  Math Function1 : Math  SaturateOnIntegerOverflow=on
  Math Function2 : Math  SaturateOnIntegerOverflow=on
  Math Function3 : Math  SaturateOnIntegerOverflow=on
  Np1 : Constant
  Ns1 : Constant  Value=48
  Rp : Constant  Value=340
  Rs : Constant  Value=0.34
  Temperature : Constant  Value=25+273.15
  Voc : Constant  Value=28.6
  cells : Constant  Value=48
  k : Constant  Value=1.38e-23
  n1 : Constant  Value=1.32
  q : Constant  Value=1.6e-19
  I : Outport
  wires:
  Temperature/1 -> [Tref]
  Voc/1 -> [Voc]
  q/1 -> [q]
  Isc/1 -> [Isc]
  k/1 -> [k]
  n1/1 -> [n]
  [k] -> Divide/1
  [Top] -> Divide/2
  [q] -> Divide/3
  Divide/1 -> [Vt]
  Divide3/1 -> [Is]
  [Ish] -> Add6/2
  Add6/1 -> I/1, [I]
  [I] -> Divide8/1
  [Rs] -> Divide8/2
  Divide8/1 -> Add3/2
  [n] -> Divide9/1
  [Vt] -> Divide9/2
  Divide9/1 -> Divide6/2
  Add3/1 -> Divide6/1
  Divide6/1 -> Math Function2/1
  Math Function2/1 -> Add4/1
  Add4/1 -> Divide13/1
  [Is] -> Divide13/2
  Divide13/1 -> [Id]
  Divide4/1 -> Add1/2
  Add1/1 -> Divide5/1
  [Rp] -> Divide5/2
  Divide5/1 -> [Ish]
  [Rs] -> Divide4/2
  [I] -> Divide4/1
  KI/1 -> [KI]
  Eg./1 -> [Eg]
  [V] -> Add1/1
  [Np] -> Divide13/3
  [Iph] -> Divide12/1
  [Np] -> Divide12/2
  Divide12/1 -> Add6/1
  [Isc] -> Add5/1
  [Top] -> Add10/1
  [Tref] -> Add10/2
  Add10/1 -> Divide14/2
  [KI] -> Divide14/1
  [Voc] -> Divide17/1
  [q] -> Divide17/2
  [k] -> Divide18/1
  [C] -> Divide18/2
  [Top] -> Divide18/3
  [n] -> Divide18/4
  Divide17/1 -> Divide19/1
  Divide18/1 -> Divide19/2
  Divide19/1 -> Math Function1/1
  Constant1/1 -> Add11/2
  Math Function1/1 -> Add11/1
  Add11/1 -> Divide16/2
  Divide16/1 -> [Irs]
  [Tref] -> Divide20/2
  [Top] -> Divide20/1
  Divide20/1 -> Divide21/2, Divide21/1, Divide21/3
  Divide21/1 -> Divide22/2
  [Irs] -> Divide22/1
  [q] -> Divide23/1
  Divide23/1 -> Divide24/1
  [k] -> Divide25/1
  [n] -> Divide25/2
  Divide25/1 -> Divide24/2
  Constant5/1 -> Divide26/1
  [Top] -> Divide26/2
  Constant6/1 -> Divide27/1
  [Tref] -> Divide27/2
  Divide27/1 -> Add12/1
  Divide26/1 -> Add12/2
  Add12/1 -> Divide28/1
  Divide24/1 -> Divide28/2
  Divide28/1 -> Math Function3/1
  Divide29/1 -> Add3/1
  [Ns] -> Divide29/2
  [V] -> Divide29/1
  [Ns] -> Divide8/3
  Divide14/1 -> Add5/2
  Add5/1 -> Divide15/2
  Divide15/1 -> [Iph]
  V/1 -> [V]
  G/1 -> [Irr]
  Top/1 -> [Topp]
  cells/1 -> [C]
  [Id] -> Add6/3
  Cte/1 -> Add2/2
  Add2/1 -> [Top]
  [Topp] -> Add2/1
  [Irr] -> Divide1/1
  [Iroo] -> Divide1/2
  Divide1/1 -> Divide15/1
  Iro2/1 -> [Iroo]
  Rs/1 -> [Rs]
  Rp/1 -> [Rp]
  Ns1/1 -> [Ns]
  Np1/1 -> [Np]
  Constant3/1 -> Add4/2
  [Isc] -> Divide16/1
  Math Function3/1 -> Divide3/1
  Divide22/1 -> Divide3/2
  [Eg] -> Divide23/2

== system ugrid_hdetail_mod_linea_transmision/1Ph_Inverter_bio/Subsystem/Steper1 ==
  In1 : Inport
  Product : Product
  Step : Step  Time=st_time  SampleTime=samp_f
  Out1 : Outport
  wires:
  Step/1 -> Product/2
  In1/1 -> Product/1
  Product/1 -> Out1/1

== system ugrid_hdetail_mod_linea_transmision/1Ph_Inverter_bio/Subsystem/Steper3 ==
  In1 : Inport
  Product : Product
  Step : Step  Time=st_time  SampleTime=samp_f
  Out1 : Outport
  wires:
  Product/1 -> Out1/1
  In1/1 -> Product/1
  Step/1 -> Product/2

== system ugrid_hdetail_mod_linea_transmision/1Ph_Inverter_diesel/Subsystem/Steper1 ==
  In1 : Inport
  Product : Product
  Step : Step  Time=st_time  SampleTime=samp_f
  Out1 : Outport
  wires:
  Product/1 -> Out1/1
  In1/1 -> Product/1
  Step/1 -> Product/2

== system ugrid_hdetail_mod_linea_transmision/1Ph_Inverter_diesel/Subsystem/Steper3 ==
  In1 : Inport
  Product : Product
  Step : Step  Time=st_time  SampleTime=samp_f
  Out1 : Outport
  wires:
  Step/1 -> Product/2
  In1/1 -> Product/1
  Product/1 -> Out1/1

== system ugrid_hdetail_mod_linea_transmision/CSI_Control_BIO/PR Controller_0_ref 3/Steper6 ==
  In1 : Inport
  Product : Product
  Step : Step  Time=st_time  SampleTime=0
  Out1 : Outport
  wires:
  Product/1 -> Out1/1
  In1/1 -> Product/1
  Step/1 -> Product/2

== system ugrid_hdetail_mod_linea_transmision/CSI_Control_DIESEL/PR Controller_0_ref 3/Steper6 ==
  In1 : Inport
  Product : Product
  Step : Step  Time=st_time  SampleTime=0
  Out1 : Outport
  wires:
  Step/1 -> Product/2
  In1/1 -> Product/1
  Product/1 -> Out1/1

== matlab function ugrid_hdetail_mod_linea_transmision/1Ph_Inverter_diesel/Subsystem/not_pwm ==
  data: u input; y output
function y = fcn(u)
%#codegen

if(u==0 || u<0)
    a=15;
else
    a=0;
end;

y = a;

== matlab function ugrid_hdetail_mod_linea_transmision/1Ph_Inverter_bio/Subsystem/not_pwm ==
  data: u input; y output
function y = fcn(u)
%#codegen

if(u==0 || u<0)
    a=15;
else
    a=0;
end;

y = a;

== matlab function ugrid_hdetail_mod_linea_transmision/CSI_Control_BIO/PQ_singlePhase ==
  data: va input; p output; vb input; ia input; ib input; q output
function [p, q] = fcn(va, vb, ia, ib)
% Esta funcion calcula la potencia activa y reactiva instantanea
% para el caso mnosofasico. En la revision de 2 papers he observado
% que una manera de extender la teoria de potencia al caso monofasico
% es asumiendo la tension o corriente de una fase como la componente
% alpha y hacer un desfase de 90 grados para obtener una version
% artificial de beta.

paux=va*ia+vb*ib;
if(paux > 20e4)
    paux = 20e4;
end
if(paux < -20e4)
    paux = -20e-4;
end

p = paux/2; % potencia activa instantanea

qaux = vb*ia-va*ib;

if(qaux>20e4)
    qaux=20e4;
end
if(qaux<-20e4)
    qaux=-20e4;
end

q = qaux/2; % potencia reactiva instantanea

== matlab function ugrid_hdetail_mod_linea_transmision/CSI_Control_DIESEL/PQ2AlphBetaCurrents_SinglePhase ==
  data: Va input; Ia output; Vb input; p input; q input; Ib output
function [Ia, Ib] = fcn(Va, Vb, p, q)
%#codegen

% divide by zero protection
if(abs((Va^2+Vb^2))<=1000*eps(0))
    det = 1/eps(0);
else
    det = 1/(Va^2+Vb^2); % constante auxiliar
end;
%det = 1/(Va^2+Vb^2);

Mat = det*[Va Vb; Vb -Va];
Iab = Mat*[2*p;2*q];

Iaaux = Iab(1);
Ibaux = Iab(2);

ilim=1e3;

if(Iaaux>ilim)
    Iaaux=ilim;
end;
if(Iaaux<-ilim)
    Iaaux =-ilim;    
end;

if(isnan(Iaaux))
    Iaaux=0;
end;
%-----------------


if(Ibaux>ilim)
    Ibaux=ilim;
end;
if(Ibaux<-ilim)
    Ibaux =-ilim;    
end;

if(isnan(Ibaux))
    Ibaux=0;
end;
%-----------------


Ia = Iaaux;
Ib = Ibaux;

== matlab function ugrid_hdetail_mod_linea_transmision/CSI_Control_DIESEL/PQ_singlePhase ==
  data: va input; p output; vb input; ia input; ib input; q output
function [p, q] = fcn(va, vb, ia, ib)
% Esta funcion calcula la potencia activa y reactiva instantanea
% para el caso mnosofasico. En la revision de 2 papers he observado
% que una manera de extender la teoria de potencia al caso monofasico
% es asumiendo la tension o corriente de una fase como la componente
% alpha y hacer un desfase de 90 grados para obtener una version
% artificial de beta.

paux=va*ia+vb*ib;
if(paux > 20e4)
    paux = 20e4;
end
if(paux < -20e4)
    paux = -20e-4;
end

p = paux/2; % potencia activa instantanea

qaux = vb*ia-va*ib;

if(qaux>20e4)
    qaux=20e4;
end
if(qaux<-20e4)
    qaux=-20e4;
end

q = qaux/2; % potencia reactiva instantanea

== matlab function ugrid_hdetail_mod_linea_transmision/1Ph_Inverter_bio1/not_pwm ==
  data: u input; y output
function y = fcn(u)
%#codegen

if(u==0 || u<0)
    a=15;
else
    a=0;
end;

y = a;

== matlab function ugrid_hdetail_mod_linea_transmision/LinearProg ==
  data: P_load input; Pbo output; P_e_alt input; kb input; kd input; PdMax input; PbMax input; Pdo output; P_e_alt_min input
function [Pbo, Pdo] = fcn(P_load, P_e_alt, kb, kd, PdMax, PbMax, P_e_alt_min)

% P_load es la potencia que se requiere en la carga.

% P_e_alt es la potencia estimada de generacion de las energias
% alternativas

% kb y kd son los pesos de las funcion de costo.

% las salidas son las potencias optimas para bio y diesel

Pb=0;
Pd=0;

D_P_e_alt = P_e_alt - P_e_alt_min; % superaavit de energia alternativa.

flagDelt = 0;

if(D_P_e_alt >= P_load)
    flagDelt = 1;
end
   

if(flagDelt==0)
    P_trad = P_load - D_P_e_alt;
    % flag: variable que indica si tiene sentido evaluar los
    % if's que se encuentran mas adelante. es decir, si flag = 0 
    % despues del primer if entonces NO se le esta pidiendo al sistema
    % mas potencia de la que puede generar y portanto el problema de 
    % optimizacion lineal tiene sentido.
    % entonces 
    flag=0;

    if(P_trad>PdMax+PbMax)
        Pd=PdMax;
        Pb=PbMax;
        flag=1;
    end

    % si ambas energias tienen el mismo factor de costo.
    if(kd==kb && flag==0)
        Pb=P_trad/2;
        Pd=P_trad/2;
    end

    % si la energia diesel es mas cara que la biomasa.
    if(kd>kb && flag==0)
        if(P_trad<=PbMax)
            Pb=P_trad;
            Pd=0;
        else
            Pb=PbMax;
            Pd=P_trad-PbMax;
        end
    end

    % si la biomasa es mas cara que la diesel.
    if(kd<kb && flag==0)
        if(P_trad<=PdMax)
            Pd=P_trad;
            Pb=0;
        else
            Pd=PdMax;
            Pb=P_trad-PdMax;
        end
    end
end

Pbo=Pb;
Pdo=Pd;

== matlab function ugrid_hdetail_mod_linea_transmision/CSI_Control_BIO/PQ2AlphBetaCurrents_SinglePhase ==
  data: Va input; Ia output; Vb input; p input; q input; Ib output
function [Ia, Ib] = fcn(Va, Vb, p, q)
%#codegen

% divide by zero protection
if(abs((Va^2+Vb^2))<=1000*eps(0))
    det = 1/eps(0);
else
    det = 1/(Va^2+Vb^2); % constante auxiliar
end;
%det = 1/(Va^2+Vb^2);

Mat = det*[Va Vb; Vb -Va];
Iab = Mat*[2*p;2*q];

Iaaux = Iab(1);
Ibaux = Iab(2);

ilim=1e3;

if(Iaaux>ilim)
    Iaaux=ilim;
end;
if(Iaaux<-ilim)
    Iaaux =-ilim;    
end;

if(isnan(Iaaux))
    Iaaux=0;
end;
%-----------------


if(Ibaux>ilim)
    Ibaux=ilim;
end;
if(Ibaux<-ilim)
    Ibaux =-ilim;    
end;

if(isnan(Ibaux))
    Ibaux=0;
end;
%-----------------


Ia = Iaaux;
Ib = Ibaux;

== matlab function ugrid_hdetail_mod_linea_transmision/LinearProg1 ==
  data: Q_load input; Qbo output; Q_e_alt input; kb input; kd input; QdMax input; QbMax input; Qdo output; Q_e_alt_min input
function [Qbo, Qdo] = fcn(Q_load, Q_e_alt, kb, kd, QdMax, QbMax, Q_e_alt_min)

% Q_load es la Qotencia que se requiere en la carga.

% Q_e_alt es la Qotencia estimada de generacion de las energias
% alternativas

% kb y kd son los Qesos de las funcion de costo.

% las salidas son las Qotencias oQtimas Qara bio y diesel

Qb=0;
Qd=0;

D_Q_e_alt = Q_e_alt - Q_e_alt_min; % suQeraavit de energia alternativa.

flagDelt = 0;

if(D_Q_e_alt >= Q_load)
    flagDelt = 1;
end
   

if(flagDelt==0)
    Q_trad = Q_load - D_Q_e_alt;
    % flag: variable que indica si tiene sentido evaluar los
    % if's que se encuentran mas adelante. es decir, si flag = 0 
    % desQues del Qrimer if entonces NO se le esta Qidiendo al sistema
    % mas Qotencia de la que Quede generar y Qortanto el Qroblema de 
    % oQtimizacion lineal tiene sentido.
    % entonces 
    flag=0;

    if(Q_trad>QdMax+QbMax)
        Qd=QdMax;
        Qb=QbMax;
        flag=1;
    end

    % si ambas energias tienen el mismo factor de costo.
    if(kd==kb && flag==0)
        Qb=Q_trad/2;
        Qd=Q_trad/2;
    end

    % si la energia diesel es mas cara que la biomasa.
    if(kd>kb && flag==0)
        if(Q_trad<=QbMax)
            Qb=Q_trad;
            Qd=0;
        else
            Qb=QbMax;
            Qd=Q_trad-QbMax;
        end
    end

    % si la biomasa es mas cara que la diesel.
    if(kd<kb && flag==0)
        if(Q_trad<=QdMax)
            Qd=Q_trad;
            Qb=0;
        else
            Qd=QdMax;
            Qb=Q_trad-QdMax;
        end
    end
end

Qbo=Qb;
Qdo=Qd;

== matlab function ugrid_hdetail_mod_linea_transmision/MATLAB Function1 ==
  data: SOC input; MaxP output; MaxQ output
function [MaxP, MaxQ] = fcn(SOC)


%  funcion que calcula la potencia maxima que puede suministrar las fuentes
%  renovables deacuerdo a la cantidad de carga que hay almancenada en la
%  bateria. esta va de 0 a 100%


% estoc valores que aparecen a continuacion se pusieron de manera
% arbitraria. corresponde a una persona con especialidad en la parte de
% potencia electrica determinar el verdadero algoritmo para hallar la
% potencia que deberia suministrar el nodo de energia renovable deacuerdo a
% la carga de la bateria.

MaxP = 0;
MaxQ = 0;

if( SOC >= 90 )
    MaxP = 500;
    MaxQ = 5000;
end

if( SOC <= 90 )
    MaxP = 200;
    MaxQ = 4000;
end

if( SOC <= 70 )
    MaxP = 100;
    MaxQ = 1000;
end

if( SOC <= 60 )
    MaxP = 50;
    MaxQ = 500;
end

== matlab function ugrid_hdetail_mod_linea_transmision/generador biomasa/MATLAB Function ==
  data: u1 input; y output; u2 input
function y = fcn(u1,u2)

y = u2*(1-u1);

== matlab function ugrid_hdetail_mod_linea_transmision/generador biomasa/MATLAB Function Acetogenesis ==
  data: Xacid input; b input; V input; Ffeed input; um input; Kd input; Ks input; Xacidp output; Sb input
function Xacidp = fcn(Xacid,b,V,Ffeed,um,Kd,Ks,Sb)

% Xacidp=(um/(1+Ks/Sb)-Kd-Ffeed/(b*V))*Xacid;
Xacidp=(um/(Ks/(1+Sb))-Kd-Ffeed/(b*V))*Xacid;

== matlab function ugrid_hdetail_mod_linea_transmision/generador biomasa/MATLAB Function Acidogenesis ==
  data: Svin input; Sv input; V input; Ffeed input; um input; umc input; K2 input; K3 input; Xacid input; Xmeth input; Ks input; Svp output; Sb input; Ksc input
function Svp = fcn(Svin,Sv,V,Ffeed,um,umc,K2,K3,Xacid,Xmeth,Ks,Sb,Ksc)

% Svp=(Svin-Sv)*(Ffeed/V)+um*K2*Xacid/(1+Ks/Sb)-umc*K3*Xmeth/(1+Ksc/Sv);
Svp=(Svin-Sv)*(Ffeed/V)+um*K2*Xacid/(Ks/(1+Sb))-umc*K3*Xmeth/(Ksc/(1+Sv));

== matlab function ugrid_hdetail_mod_linea_transmision/generador biomasa/MATLAB Function Hidrolisis ==
  data: Sbin input; Sbp output; Sb input; V input; Ffeed input; um input; K1 input; Xacid input; Ks input
function Sbp = fcn(Sbin,Sb,V,Ffeed,um,K1,Xacid,Ks)

% Sbp=(Sbin-Sb)*(Ffeed/V)+um*K1*Xacid/(1+Ks/Sb);
Sbp=(Sbin-Sb)*(Ffeed/V)+um*K1*Xacid/(Ks/(1+Sb));

== matlab function ugrid_hdetail_mod_linea_transmision/generador biomasa/MATLAB Function metano ==
  data: Xmeth input; K4 input; V input; umc input; Ksc input; Sv input; Fmeth output
function Fmeth = fcn(Xmeth,K4,V,umc,Ksc,Sv)


% Fmeth=V*umc*K4*Xmeth/(Ksc/Sv+1);
Fmeth=V*umc*K4*Xmeth/(Ksc/(Sv+1));

== matlab function ugrid_hdetail_mod_linea_transmision/generador biomasa/MATLAB Function metanogenesis ==
  data: Xmeth input; b input; V input; Ffeed input; umc input; Ksc input; Sv input; Xmethp output; Kdc input
function Xmethp = fcn(Xmeth,b,V,Ffeed,umc,Ksc,Sv,Kdc)

% Xmethp=(umc/(Ksc/Sv+1)-Kdc-Ffeed/(b*V))*Xmeth;
Xmethp=(umc/(Ksc/(Sv+1))-Kdc-Ffeed/(b*V))*Xmeth;
